simulink model "quadXmodel"  (R2018b)
settings: Solver=ode1  StartTime=0.0  StopTime=tfinal  FixedStep=dt  RelTol=1e-3
values from neighbouring files (symbols this model uses):
  g = [0 0 9.81]'    [quadSimRunMain.m]    (also in quadSymbolicCalculation.m = [0 0 sym('g','real')]'; quadVisualizationManager.m = quiver(X,Y,U,V); quadtrapezoidal.m = 9.81; runquadXModel.m = 9.81)
  lambda = 0.36    [runquadXModel.m]
undefined symbols (not defined in the file or in its folder): ad2, bd2, DiscIntNeverNeededParam
libraries: simulink x1
settings Model: Creator=duho46  LastModifiedBy=duho46

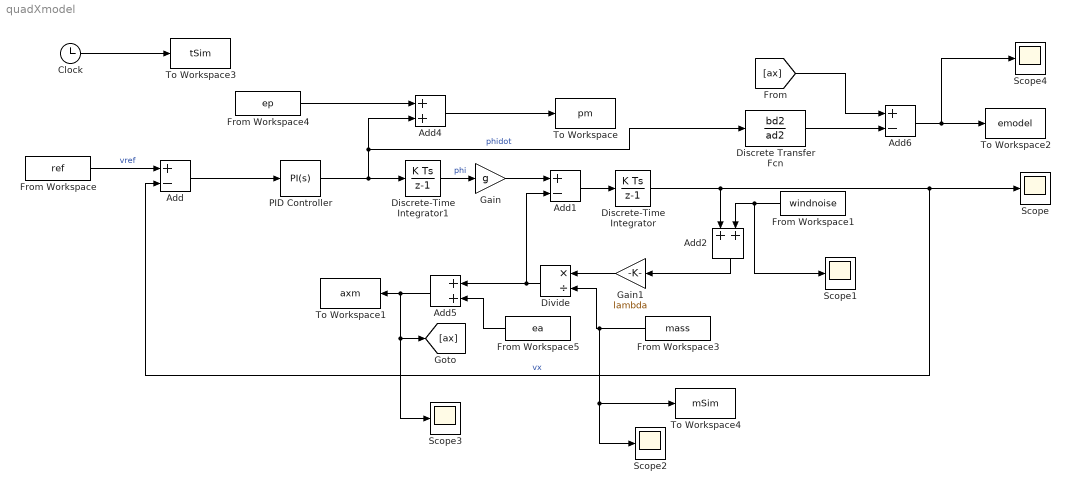
== system quadXmodel ==
  Add : Sum  Inputs=+-
  Add1 : Sum  Inputs=+-
  Add2 : Sum
  Add4 : Sum
  Add5 : Sum
  Add6 : Sum  Inputs=+-
  Clock : Clock
  Discrete Transfer Fcn : DiscreteTransferFcn  Numerator=bd2  Denominator=ad2
  Discrete-Time Integrator : DiscreteIntegrator  SampleTime=-1  ICPrevOutput=DiscIntNeverNeededParam  ICPrevScaledInput=DiscIntNeverNeededParam
  Discrete-Time Integrator1 : DiscreteIntegrator  SampleTime=-1  ICPrevOutput=DiscIntNeverNeededParam  ICPrevScaledInput=DiscIntNeverNeededParam
  Divide : Product  Inputs=*/
  From Workspace : FromWorkspace  VariableName=ref  SampleTime=0
  From Workspace1 : FromWorkspace  VariableName=windnoise  SampleTime=0
  From Workspace3 : FromWorkspace  VariableName=mass  SampleTime=0
  From Workspace4 : FromWorkspace  VariableName=ep  SampleTime=0
  From Workspace5 : FromWorkspace  VariableName=ea  SampleTime=0
  Gain : Gain  Gain=g
  Gain1 : Gain  Gain=lambda
  PID Controller : simulink/Continuous/PID Controller  Controller=PI  Form=Parallel  TimeDomain=Continuous-time  SampleTime=-1  IntegratorMethod=Forward Euler  FilterMethod=Forward Euler  ControllerParametersSource=internal  P=1  I=0.1  D=0  UseFilter=on  N=100  TunerSelectOption=Transfer Function Based (PID Tuner App)  InitialConditionSource=internal  InitialConditionForIntegrator=0  InitialConditionForFilter=0  DifferentiatorICPrevScaledInput=0  ExternalReset=none  TrackingMode=off  Kt=1  LimitOutput=off  UpperSaturationLimit=inf  LowerSaturationLimit=-inf  LinearizeAsGain=on  AntiWindupMode=none  Kb=1  POutMin=[]  POutMax=[]  IOutMin=[]  IOutMax=[]  DOutMin=[]  DOutMax=[]  NOutMin=[]  NOutMax=[]  SumOutMin=[]  SumOutMax=[]  SaturationOutMin=[]  SaturationOutMax=[]  PParamMin=[]  PParamMax=[]  IParamMin=[]  IParamMax=[]  DParamMin=[]  DParamMax=[]  NParamMin=[]  NParamMax=[]  KbParamMin=[]  KbParamMax=[]  KtParamMin=[]  KtParamMax=[]  KbOutMin=[]  KbOutMax=[]  KtOutMin=[]  KtOutMax=[]  IntegratorOutMin=[]  IntegratorOutMax=[]  FilterOutMin=[]  FilterOutMax=[]  SumI1OutMin=[]  SumI1OutMax=[]  SumI2OutMin=[]  SumI2OutMax=[]  SumI3OutMin=[]  SumI3OutMax=[]  SumI4OutMin=[]  SumI4OutMax=[]  SumDOutMin=[]  SumDOutMax=[]  DifferentiatorOutMin=[]  DifferentiatorOutMax=[]  FilterDiffOutCoefMin=[]  FilterDiffOutCoefMax=[]  ReciprocalOutMin=[]  ReciprocalOutMax=[]  SumDenOutMin=[]  SumDenOutMax=[]  SumNumOutMin=[]  SumNumOutMax=[]  DivideOutMin=[]  DivideOutMax=[]  IntegratorContinuousStateAttributes=''  IntegratorStateMustResolveToSignalObject=off  IntegratorRTWStateStorageClass=Auto  FilterContinuousStateAttributes=''  FilterStateMustResolveToSignalObject=off  FilterRTWStateStorageClass=Auto  ParallelPVariant=InternalParameters  IdealPVariant=Disabled  IVariant=InternalParameters  DVariant=Disabled  IntegratorVariant=Continuous  SatVariant=Disabled  AWVariant=Passthrough  PCopyVariant=Disabled  TRVariant=Disabled  FdbkBlocksVariant=Forward  IdealPFdbkVariant=Disabled  SatFdbkVariant=Disabled  DerivativeFilterVariant=Disabled  NVariant=Disabled  NCopyVariant=Disabled_SignalSpec  FilterICVariant=Disabled  IntegratorICVariant=InternalICs  ExternalResetVariant=Disabled  TRSumVariant=Passthrough  SumFdbkVariant=Disabled  SumVariant=Sum_PI
  Scope{,1..4} (5 alike) : Scope
  To Workspace : ToWorkspace  VariableName=pm  SampleTime=-1
  To Workspace1 : ToWorkspace  VariableName=axm  SampleTime=-1
  To Workspace2 : ToWorkspace  VariableName=emodel  SampleTime=-1
  To Workspace3 : ToWorkspace  VariableName=tSim  SampleTime=-1
  To Workspace4 : ToWorkspace  VariableName=mSim  SampleTime=-1
  wires:
  From Workspace/1 -> Add/1  "vref"
  Add/1 -> PID Controller/1
  Discrete-Time Integrator1/1 -> Gain/1  "phi"
  Gain/1 -> Add1/1
  Add1/1 -> Discrete-Time Integrator/1
  Discrete-Time Integrator/1 -> Scope/1, Add/2, Add2/1  "vx"
  Gain1/1 -> Divide/1
  Divide/1 -> Add5/1, Add1/2
  From Workspace3/1 -> To Workspace4/1, Scope2/1, Divide/2
  Add2/1 -> Gain1/1
  From Workspace1/1 -> Scope1/1, Add2/2
  From Workspace4/1 -> Add4/1
  Add4/1 -> To Workspace/1
  From Workspace5/1 -> Add5/2
  Add5/1 -> [ax], Scope3/1, To Workspace1/1
  PID Controller/1 -> Discrete-Time Integrator1/1, Discrete Transfer Fcn/1, Add4/2  "phidot"
  Discrete Transfer Fcn/1 -> Add6/2
  [ax] -> Add6/1
  Add6/1 -> Scope4/1, To Workspace2/1
  Clock/1 -> To Workspace3/1
